simulink model "LIDAR"  (R2020b)
settings: Solver=FixedStepAuto  StartTime=0.0  StopTime=10.0  FixedStep=DT  RelTol=1e-3
undefined symbols (not defined in the file or in its folder): LIDAR_phi0, PR_A, PR_B, PR_C, PR_L, PR_theta0
settings Model: Creator=lpwoolcock  LastModifiedBy=lpwoolcock

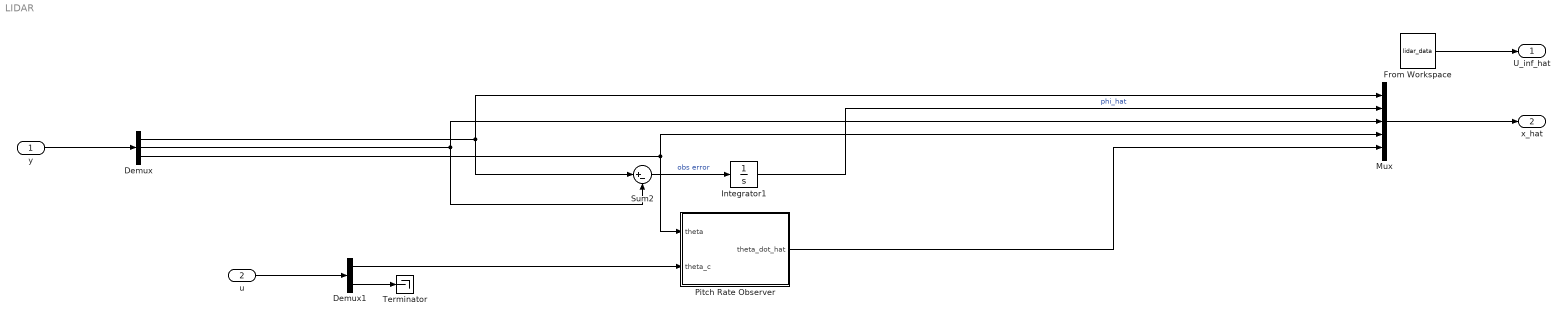
== system LIDAR ==
  y : Inport  PortDimensions=[3 1]
  u : Inport  Port=2  PortDimensions=[2 1]
  Demux : Demux  Outputs=3
  Demux1 : Demux  Outputs=2
  From Workspace : FromWorkspace  VariableName=lidar_data
  Integrator1 : Integrator  InitialCondition=LIDAR_phi0
  Mux : Mux  Inputs=5
  Pitch Rate Observer : Subsystem  TreatAsAtomicUnit=on
  Sum2 : Sum  Inputs=|+-
  Terminator : Terminator
  U_inf_hat : Outport  PortDimensions=1
  x_hat : Outport  Port=2  PortDimensions=[5 1]
  wires:
  Sum2/1 -> Integrator1/1  "obs error"
  Demux/3 -> Pitch Rate Observer/1(theta), Mux/4
  Integrator1/1 -> Mux/2  "phi_hat"
  Demux/1 -> Mux/1, Sum2/1
  Demux/2 -> Mux/3, Sum2/2
  Demux1/1 -> Pitch Rate Observer/2(theta_c)
  y/1 -> Demux/1
  u/1 -> Demux1/1
  Mux/1 -> x_hat/1
  From Workspace/1 -> U_inf_hat/1
  Pitch Rate Observer/1(theta_dot_hat) -> Mux/5
  Demux1/2 -> Terminator/1

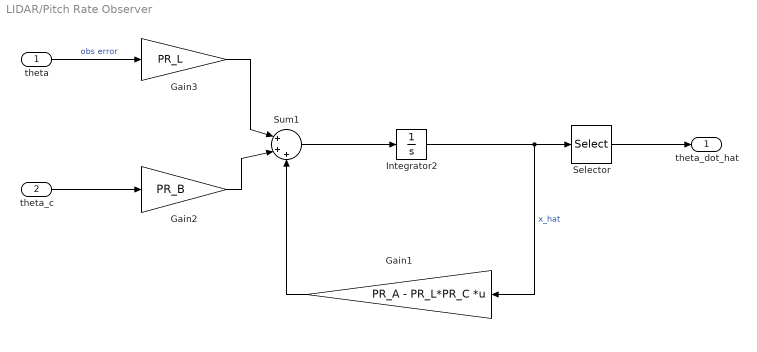
== system LIDAR/Pitch Rate Observer ==
  theta : Inport
  theta_c : Inport  Port=2
  Gain1 : Gain  Gain=PR_A - PR_L*PR_C  Multiplication=Matrix(K*u)
  Gain2 : Gain  Gain=PR_B
  Gain3 : Gain  Gain=PR_L
  Integrator2 : Integrator  InitialCondition=PR_theta0
  Selector : Selector  InputPortWidth=2  IndexOptions=Index vector (dialog)  Indices=[2]  OutputSizes=1
  Sum1 : Sum  Inputs=|+++
  theta_dot_hat : Outport
  wires:
  Sum1/1 -> Integrator2/1
  Gain2/1 -> Sum1/2
  Gain3/1 -> Sum1/1
  Integrator2/1 -> Selector/1, Gain1/1  "x_hat"
  theta/1 -> Gain3/1  "obs error"
  Gain1/1 -> Sum1/3
  theta_c/1 -> Gain2/1
  Selector/1 -> theta_dot_hat/1
